simulink model "modelZWoda"  (R2015a)
settings: Solver=ode4  StartTime=0.0  StopTime=T_sim  FixedStep=0.01  RelTol=1e-3
values from neighbouring files (symbols this model uses):
  I = Nastawy(2)    [LP1.m]    (also in USImodel.m; opt_pid.m = input(2); parametryPID.m = 0.88; wskaJak1.m = params(2))
  J2 = Jr + mw * r*r    (= 0.541666666667)    [LP1.m]    (also in ParametryDoSymulacji.m; USImodel.m; wskaJak1.m; wskaJak2.m)
  k = 0.1    [LP1.m]    (also in ParametryDoSymulacji.m; USImodel.m; wskaJak1.m; wskaJak2.m)
  ke = 5    [LP1.m]    (also in ParametryDoSymulacji.m; USImodel.m; wskaJak1.m; wskaJak2.m)
  L = 0.1    [LP1.m]    (also in ParametryDoSymulacji.m; USImodel.m; wskaJak1.m; wskaJak2.m)
  P = Nastawy(1)    [LP1.m]    (also in USImodel.m; opt_pid.m = input(1); parametryPID.m = 1.5; wskaJak1.m = params(1))
  R = 2    [LP1.m]    (also in ParametryDoSymulacji.m; USImodel.m; wskaJak1.m; wskaJak2.m)
libraries: simulink x1
settings Model: Creator=Kamil  LastModifiedBy=Kamil

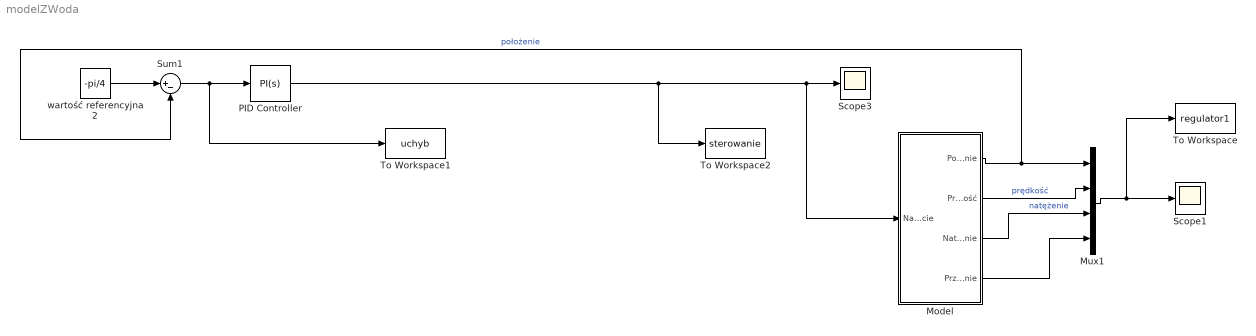
== system modelZWoda ==
  Model : Subsystem
  Mux1 : Mux
  PID Controller : simulink/Continuous/PID Controller  Controller=PI  TimeDomain=Continuous-time  SampleTime=-1  IntegratorMethod=Forward Euler  FilterMethod=Forward Euler  Form=Ideal  UseFilter=on  ControllerParametersSource=internal  P=P  I=I  D=0  N=100  InitialConditionSource=internal  InitialConditionForIntegrator=0  InitialConditionForFilter=0  ExternalReset=none  LimitOutput=off  UpperSaturationLimit=inf  LowerSaturationLimit=-inf  LinearizeAsGain=on  AntiWindupMode=none  Kb=1  TrackingMode=off  Kt=1  PParamMin=[]  PParamMax=[]  IParamMin=[]  IParamMax=[]  DParamMin=[]  DParamMax=[]  NParamMin=[]  NParamMax=[]  KbParamMin=[]  KbParamMax=[]  KtParamMin=[]  KtParamMax=[]  POutMin=[]  POutMax=[]  IOutMin=[]  IOutMax=[]  DOutMin=[]  DOutMax=[]  NOutMin=[]  NOutMax=[]  KbOutMin=[]  KbOutMax=[]  KtOutMin=[]  KtOutMax=[]  IntegratorOutMin=[]  IntegratorOutMax=[]  FilterOutMin=[]  FilterOutMax=[]  SumOutMin=[]  SumOutMax=[]  SumI1OutMin=[]  SumI1OutMax=[]  SumI2OutMin=[]  SumI2OutMax=[]  SumI3OutMin=[]  SumI3OutMax=[]  SumDOutMin=[]  SumDOutMax=[]  SaturationOutMin=[]  SaturationOutMax=[]  IntegratorContinuousStateAttributes=''  IntegratorStateMustResolveToSignalObject=off  IntegratorRTWStateStorageClass=Auto  FilterContinuousStateAttributes=''  FilterStateMustResolveToSignalObject=off  FilterRTWStateStorageClass=Auto  DifferentiatorICPrevScaledInput=0  DifferentiatorOutMin=[]  DifferentiatorOutMax=[]
  Scope1 : Scope
      settings: TimeRange=50  YMin=-1  YMax=0.8  MaxDataPoints=10000
  Scope3 : Scope
      settings: SaveName=ScopeData3
  Sum1 : Sum  Inputs=|+-
  To Workspace : ToWorkspace  VariableName=regulator1  SaveFormat=Structure With Time  SampleTime=-1
  To Workspace1 : ToWorkspace  VariableName=uchyb  SaveFormat=Structure With Time  SampleTime=-1
  To Workspace2 : ToWorkspace  VariableName=sterowanie  SaveFormat=Structure With Time  SampleTime=-1
  wartość referencyjna 2 : Constant  Value=-pi/4
  wires:
  wartość referencyjna 2/1 -> Sum1/1
  PID Controller/1 -> To Workspace2/1, Model/1(Napięcie), Scope3/1
  Model/1(Położenie) -> Sum1/2, Mux1/1  "położenie"
  Model/3("Natężenie ") -> Mux1/3  "natężenie"
  Model/2(Prędkość) -> Mux1/2  "prędkość"
  Mux1/1 -> To Workspace/1, Scope1/1
  Sum1/1 -> To Workspace1/1, PID Controller/1
  Model/4("Przyspieszenie ") -> Mux1/4

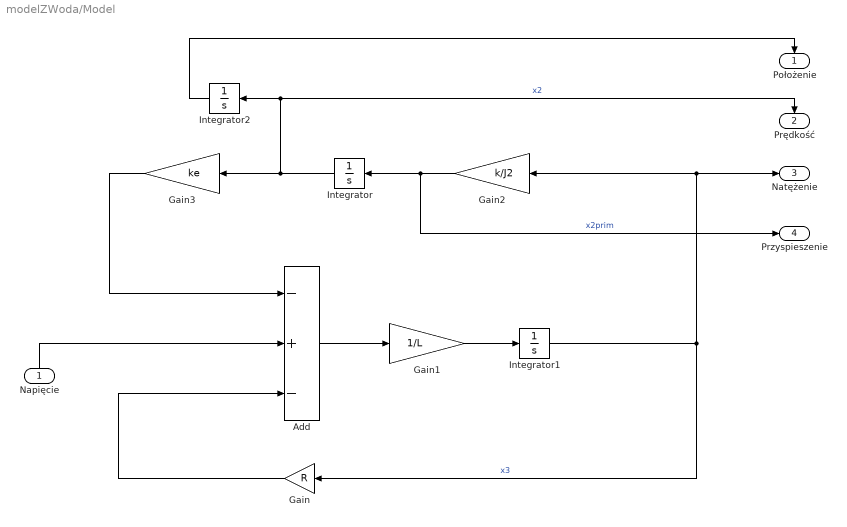
== system modelZWoda/Model ==
  Napięcie : Inport
  Add : Sum  Inputs=-+-
  Gain : Gain  Gain=R
  Gain1 : Gain  Gain=1/L
  Gain2 : Gain  Gain=k/J2
  Gain3 : Gain  Gain=ke
  Integrator : Integrator
  Integrator1 : Integrator
  Integrator2 : Integrator  InitialCondition=pi/4
  Położenie : Outport
  Prędkość : Outport  Port=2
  "Natężenie " : Outport  Port=3
  "Przyspieszenie " : Outport  Port=4
  wires:
  Add/1 -> Gain1/1
  Gain1/1 -> Integrator1/1
  Gain3/1 -> Add/1
  Integrator/1 -> Prędkość/1, Integrator2/1, Gain3/1  "x2"
  Integrator2/1 -> Położenie/1
  Gain/1 -> Add/3
  Integrator1/1 -> "Natężenie "/1, Gain2/1, Gain/1  "x3"
  Gain2/1 -> "Przyspieszenie "/1, Integrator/1  "x2prim"
  Napięcie/1 -> Add/2
